simulink model "ZiglerNicholsBTVNCONGA1"  (R2014a)
settings: Solver=ode45  StartTime=0.0  StopTime=10.0  RelTol=1e-3
undefined symbols (not defined in the file or in its folder): i
settings Model: Creator=tri  LastModifiedBy=tri

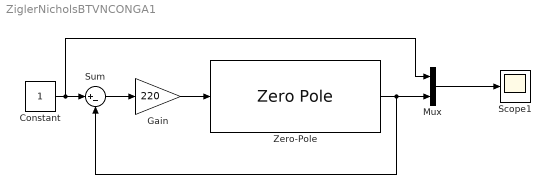
== system ZiglerNicholsBTVNCONGA1 ==
  Constant : Constant
  Gain : Gain  Gain=220
  Mux : Mux  Inputs=2
  Scope1 : Scope
  Sum : Sum  Inputs=|+-
  Zero-Pole : ZeroPole  Zeros=[]  Poles=[-5+5*(sqrt(3))*i -5-5*(sqrt(3))*i ]  Gain=100
  wires:
  Gain/1 -> Zero-Pole/1
  Zero-Pole/1 -> Sum/2, Mux/2
  Mux/1 -> Scope1/1
  Constant/1 -> Mux/1, Sum/1
  Sum/1 -> Gain/1
